simulink model "ESM_TeslaModelS_statKreisfahrt"  (R2020b)
settings: Solver=FixedStepAuto  StartTime=0.0  StopTime=StopTime  FixedStep=SampleTime  RelTol=1e-3
undefined symbols (not defined in the file): ayObs, c_alpha_F, c_alpha_R, c_alpha_rear_mean, DiscIntNeverNeededParam, I_S, init, input_r, m_vehicle, par_TIR, par_VEH, parameter, SelectManeuver, simtime, Single_Track_Model_linear, SingleTrackModel_linear
libraries: pid_lib x5, simulink x3, dspsigops x2, vehicle_model x1
(part 3 of 4)

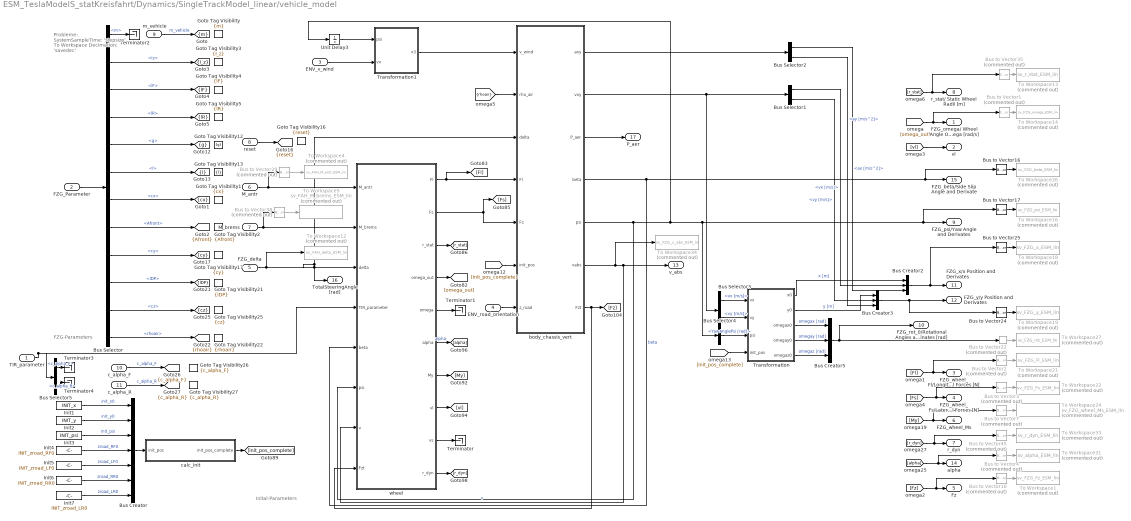
== system ESM_TeslaModelS_statKreisfahrt/Dynamics/SingleTrackModel_linear/vehicle_model ==
  note: Probleme:
      | SystemSampleTime: 'stepsize'
      |
      |
      | To Workspace
      | Decimation: 'savedec'
  note: FZG-Parameters
  note: Inital-Parameters
  TIR_parameter : Inport
  FZG_Parameter : Inport  Port=2
  ENV_v_wind : Inport  Port=3
  ENV_road_orientation : Inport  Port=4
  FZG_delta : Inport  Port=5
  M_antr : Inport  Port=6  PortDimensions=2
  M_brems : Inport  Port=7  PortDimensions=2
  reset : Inport  Port=8
  m_vehicle : Inport  Port=9
  c_alpha_F : Inport  Port=10
  c_alpha_R : Inport  Port=11
  Bus Creator : BusCreator  Inputs=7
  Bus Creator2 : BusCreator  Inputs=3
  Bus Creator3 : BusCreator  Inputs=3
  Bus Creator5 : BusCreator  Inputs=3
  Bus Selector : BusSelector  OutputSignals=m,Iz,lF,lR,g,l,cx,Afront,cy,lDP,cz,rhoair
  Bus Selector1 : BusSelector  OutputSignals=vx [m/s],vy [m/s]
  Bus Selector2 : BusSelector  OutputSignals=ax [m/s^2],ay [m/s^2]
  Bus Selector3 : BusSelector  OutputSignals=vx [m/s],vy [m/s]
  Bus Selector4 : BusSelector  OutputSignals=YawAnglePsi [rad]
  Bus Selector5 : BusSelector  OutputSignals=front.c_alpha_F,rear.c_alpha_R
  Bus to Vector{1..4,7,10,22,29,35,38,45} (11 alike) : BusToVector  Commented=on
  Bus to Vector{16..17,24..25} (4 alike) : BusToVector
  Goto Tag Visibility : GotoTagVisibility  GotoTag=m
  Goto Tag Visibility1 : GotoTagVisibility  GotoTag=cx
  Goto Tag Visibility12 : GotoTagVisibility  GotoTag=g
  Goto Tag Visibility13 : GotoTagVisibility  GotoTag=l
  Goto Tag Visibility16 : GotoTagVisibility  GotoTag=reset
  Goto Tag Visibility17 : GotoTagVisibility  GotoTag=cy
  Goto Tag Visibility2 : GotoTagVisibility  GotoTag=Afront
  Goto Tag Visibility21 : GotoTagVisibility  GotoTag=lDP
  Goto Tag Visibility22 : GotoTagVisibility  GotoTag=rhoair
  Goto Tag Visibility25 : GotoTagVisibility  GotoTag=cz
  Goto Tag Visibility26 : GotoTagVisibility  GotoTag=c_alpha_F
  Goto Tag Visibility27 : GotoTagVisibility  GotoTag=c_alpha_R
  Goto Tag Visibility3 : GotoTagVisibility  GotoTag=I_z
  Goto Tag Visibility4 : GotoTagVisibility  GotoTag=lF
  Goto Tag Visibility5 : GotoTagVisibility  GotoTag=lR
  Init1 : Constant  Value=INIT_x
  Init2 : Constant  Value=INIT_y
  Init3 : Constant  Value=INIT_psi
  Init4 : Constant  Value=INIT_zroad_RF0
  Init5 : Constant  Value=INIT_zroad_LF0
  Init6 : Constant  Value=INIT_zroad_RR0
  Init7 : Constant  Value=INIT_zroad_LR0
  Terminator{,1..4} (5 alike) : Terminator
  To Workspace1 : ToWorkspace  Commented=on  VariableName=sv_FZG_Fz_ESM_lin  SampleTime=-1
      settings: Decimation=savedec  Save2DSignal=2-D array (concatenate along first dimension)
  To Workspace12 : ToWorkspace  Commented=on  VariableName=sv_FAH_delta_ESM_lin  SampleTime=-1
      settings: Decimation=savedec  Save2DSignal=2-D array (concatenate along first dimension)
  To Workspace13 : ToWorkspace  Commented=on  VariableName=sv_r_stat_ESM_lin  SampleTime=-1
      settings: Decimation=savedec  Save2DSignal=2-D array (concatenate along first dimension)
  To Workspace14 : ToWorkspace  Commented=on  VariableName=sv_FZG_omega_ESM_lin  SampleTime=-1
      settings: Decimation=savedec  Save2DSignal=2-D array (concatenate along first dimension)
  To Workspace16 : ToWorkspace  Commented=on  VariableName=sv_FZG_psi_ESM_lin  SampleTime=-1
      settings: Decimation=savedec  Save2DSignal=2-D array (concatenate along first dimension)
  To Workspace18 : ToWorkspace  Commented=on  VariableName=sv_FZG_x_ESM_lin  SampleTime=-1
      settings: Decimation=savedec  Save2DSignal=2-D array (concatenate along first dimension)
  To Workspace19 : ToWorkspace  Commented=on  VariableName=sv_FZG_y_ESM_lin  SampleTime=-1
      settings: Decimation=savedec  Save2DSignal=2-D array (concatenate along first dimension)
  To Workspace21 : ToWorkspace  Commented=on  VariableName=sv_FZG_Fl_ESM_lin  SampleTime=-1
      settings: Decimation=savedec  Save2DSignal=2-D array (concatenate along first dimension)
  To Workspace22 : ToWorkspace  Commented=on  VariableName=sv_FZG_Fs_ESM_lin  SampleTime=-1
      settings: Decimation=savedec  Save2DSignal=2-D array (concatenate along first dimension)
  To Workspace24 : ToWorkspace  Commented=on  VariableName=sv_FZG_wheel_Ms_ESM_lin  SampleTime=-1
      settings: Decimation=savedec  Save2DSignal=2-D array (concatenate along first dimension)
  To Workspace26 : ToWorkspace  Commented=on  VariableName=sv_FZG_beta_ESM_lin  SampleTime=-1
      settings: Decimation=savedec  Save2DSignal=2-D array (concatenate along first dimension)
  To Workspace27 : ToWorkspace  Commented=on  VariableName=sv_FZG_rot_ESM_lin  SampleTime=-1
      settings: Decimation=savedec  Save2DSignal=2-D array (concatenate along first dimension)
  To Workspace31 : ToWorkspace  Commented=on  VariableName=sv_alpha_ESM_lin  SampleTime=-1
      settings: Decimation=savedec  Save2DSignal=2-D array (concatenate along first dimension)
  To Workspace33 : ToWorkspace  Commented=on  VariableName=sv_r_dyn_ESM_lin  SampleTime=-1
      settings: Decimation=savedec  Save2DSignal=2-D array (concatenate along first dimension)
  To Workspace34 : ToWorkspace  Commented=on  VariableName=sv_FZG_v_abs_ESM_lin  SampleTime=-1
      settings: Decimation=savedec  Save2DSignal=2-D array (concatenate along first dimension)
  To Workspace4 : ToWorkspace  Commented=on  VariableName=sv_FAH_M_antr_ESM_lin  SampleTime=-1
      settings: Decimation=savedec  Save2DSignal=2-D array (concatenate along first dimension)
  To Workspace5 : ToWorkspace  Commented=on  VariableName=sv_FAH_M_brems_ESM_lin  SampleTime=-1
      settings: Decimation=savedec  Save2DSignal=2-D array (concatenate along first dimension)
  Transformation : Subsystem
  Transformation1 : Subsystem
  Unit Delay3 : UnitDelay  SampleTime=-1  HasFrameUpgradeWarning=on
  body_chassis_vert : Subsystem
  calc_init : Subsystem
  wheel : Subsystem
  FZG_omega/ Wheel Angle Omega [rad/s] : Outport  VectorParamsAs1DForOutWhenUnconnected=off
  vl : Outport  Port=2  VectorParamsAs1DForOutWhenUnconnected=off
  FZG_wheel_Fl/Longitudinal Wheel Forces [N] : Outport  Port=3  VectorParamsAs1DForOutWhenUnconnected=off
  FZG_wheel_Fs/Lateral Wheel Forces [N] : Outport  Port=4  VectorParamsAs1DForOutWhenUnconnected=off
  Fz : Outport  Port=5  VectorParamsAs1DForOutWhenUnconnected=off
  FZG_wheel_Ms : Outport  Port=6  VectorParamsAs1DForOutWhenUnconnected=off
  r_dyn : Outport  Port=7  VectorParamsAs1DForOutWhenUnconnected=off
  r_stat/ Static Wheel Radii [m] : Outport  Port=8  VectorParamsAs1DForOutWhenUnconnected=off
  FZG_psi/Yaw Angle and Derivates : Outport  Port=9  VectorParamsAs1DForOutWhenUnconnected=off
  FZG_rot_0/Rotational Angles around Initial Coordinates [rad] : Outport  Port=10  VectorParamsAs1DForOutWhenUnconnected=off
  FZG_x/x Position and Derivates : Outport  Port=11  PortDimensions=3  VectorParamsAs1DForOutWhenUnconnected=off
  FZG_y/y Position and Derivates : Outport  Port=12  VectorParamsAs1DForOutWhenUnconnected=off
  v_abs : Outport  Port=13  VectorParamsAs1DForOutWhenUnconnected=off
  alpha : Outport  Port=14  VectorParamsAs1DForOutWhenUnconnected=off
  FZG_beta/Side Slip Angle and Derivate : Outport  Port=15  VectorParamsAs1DForOutWhenUnconnected=off
  TotalSteeringAngle [rad] : Outport  Port=16  VectorParamsAs1DForOutWhenUnconnected=off
  P_aer : Outport  Port=17  VectorParamsAs1DForOutWhenUnconnected=off
  tag scope: Afront=scoped, I_z=scoped, c_alpha_F=scoped, c_alpha_R=scoped, cx=scoped, cy=scoped, cz=scoped, g=scoped, l=scoped, lDP=scoped, lF=scoped, lR=scoped, m=scoped, reset=scoped, rhoair=scoped
  wires:
  M_antr/1 -> wheel/1(M_antr), Bus to Vector29/1
  Bus to Vector29/1 -> To Workspace4/1
  M_brems/1 -> Bus to Vector38/1, wheel/2(M_brems)
  Bus to Vector38/1 -> To Workspace5/1
  FZG_delta/1 -> wheel/3(delta), body_chassis_vert/3(delta), TotalSteeringAngle [rad]/1, To Workspace12/1
  Bus to Vector2/1 -> To Workspace21/1
  Bus to Vector25/1 -> To Workspace18/1
  Bus Creator5/1 -> Bus to Vector22/1, FZG_rot_0/Rotational Angles around Initial Coordinates [rad]/1
  Bus to Vector4/1 -> To Workspace31/1
  Bus to Vector1/1 -> To Workspace14/1
  Bus to Vector16/1 -> To Workspace26/1
  Bus to Vector24/1 -> To Workspace19/1
  [omega_out] -> FZG_omega/ Wheel Angle Omega [rad/s]/1, Bus to Vector1/1
  Bus to Vector17/1 -> To Workspace16/1
  Bus Creator3/1 -> Bus to Vector24/1, FZG_y/y Position and Derivates/1
  Bus to Vector3/1 -> To Workspace22/1
  Bus to Vector7/1 -> To Workspace24/1
  Bus to Vector35/1 -> To Workspace13/1
  Bus to Vector45/1 -> To Workspace33/1
  [Fl] -> FZG_wheel_Fl/Longitudinal Wheel Forces [N]/1, Bus to Vector2/1
  body_chassis_vert/5(psi) -> wheel/6(psi), Unit Delay3/1, Bus Selector4/1, FZG_psi/Yaw Angle and Derivates/1, Bus to Vector17/1
  [Fs] -> FZG_wheel_Fs/Lateral Wheel Forces [N]/1, Bus to Vector3/1
  [r_dyn] -> r_dyn/1, Bus to Vector45/1
  [My] -> FZG_wheel_Ms/1, Bus to Vector7/1
  Bus to Vector10/1 -> To Workspace1/1
  body_chassis_vert/4(beta) -> wheel/5(beta), FZG_beta/Side Slip Angle and Derivate/1, Bus to Vector16/1  "beta"
  [Fz] -> Fz/1, Bus to Vector10/1
  Bus Creator2/1 -> FZG_x/x Position and Derivates/1, Bus to Vector25/1
  [r_stat] -> r_stat/ Static Wheel Radii [m]/1, Bus to Vector35/1
  [alpha] -> alpha/1, Bus to Vector4/1
  Bus to Vector22/1 -> To Workspace27/1
  c_alpha_R/1 -> [c_alpha_R]  "c_alpha_R"
  c_alpha_F/1 -> [c_alpha_F]  "c_alpha_F"
  Init7/1 -> Bus Creator/7  "zroad_LR0"
  Init6/1 -> Bus Creator/6  "zroad_RR0"
  Init5/1 -> Bus Creator/5  "zroad_LF0"
  Init4/1 -> Bus Creator/4  "zroad_RF0"
  Init3/1 -> Bus Creator/3  "init_psi"
  Init2/1 -> Bus Creator/2  "init_y0"
  Init1/1 -> Bus Creator/1  "init_x0"
  [vl] -> vl/1
  wheel/10(r_dyn) -> [r_dyn]
  wheel/6(alpha) -> [alpha]  "alpha"
  wheel/9(vs) -> Terminator/1
  wheel/8(vl) -> [vl]
  wheel/7(My) -> [My]
  wheel/3(r_stat) -> [r_stat]
  [init_pos_complete] -> Transformation/4(init_pos)
  [init_pos_complete] -> body_chassis_vert/6(init_pos)
  calc_init/1(init_pos_complete) -> [init_pos_complete]
  TIR_parameter/1 -> wheel/4(TIR_parameter), Bus Selector5/1
  wheel/5(omega) -> Terminator1/1
  wheel/4(omega_out) -> [omega_out]
  body_chassis_vert/3(P_aer) -> P_aer/1
  Bus Selector/7 -> [cx]  "<cx>"
  Bus Selector/8 -> [Afront]  "<Afront>"
  Bus Selector/10 -> [lDP]  "<lDP>"
  Bus Selector/11 -> [cz]  "<cz>"
  body_chassis_vert/1(axy) -> Bus Selector2/1
  body_chassis_vert/2(vxy) -> Bus Selector1/1, Bus Selector3/1
  Bus Selector/9 -> [cy]  "<cy>"
  Unit Delay3/1 -> Transformation1/1(psi)
  Transformation1/1(x3) -> body_chassis_vert/1(v_wind)
  Bus Creator/1 -> calc_init/1(init_pos)
  Transformation/5(omegaz0) -> Bus Creator5/3  "omegaz [rad]"
  Transformation/4(omegay0) -> Bus Creator5/2  "omegay [rad]"
  Transformation/3(omegax0) -> Bus Creator5/1  "omegax [rad]"
  Bus Selector4/1 -> Transformation/3(psi)  "<YawAnglePsi [rad]>"
  Bus Selector3/2 -> Transformation/2(vy)  "<vy [m/s]>"
  Bus Selector3/1 -> Transformation/1(vx)  "<vx [m/s]>"
  Transformation/2(y0) -> Bus Creator3/1  "y [m]"
  Transformation/1(x0) -> Bus Creator2/1  "x [m]"
  ENV_road_orientation/1 -> body_chassis_vert/7(z_road)
  [rhoair] -> body_chassis_vert/2(rho_air)
  ENV_v_wind/1 -> Transformation1/2(vx)
  FZG_Parameter/1 -> Bus Selector/1
  wheel/2(Fs) -> body_chassis_vert/5(Fs), [Fs]
  body_chassis_vert/6(vabs) -> wheel/7(v), v_abs/1, To Workspace34/1  "v"
  Bus Selector/1 -> Terminator2/1  "<m>"
  Bus Selector/2 -> [I_z]  "<Iz>"
  Bus Selector/3 -> [lF]  "<lF>"
  Bus Selector/4 -> [lR]  "<lR>"
  Bus Selector/5 -> [g]  "<g>"
  Bus Selector/6 -> [l]  "<l>"
  wheel/1(Fl) -> body_chassis_vert/4(Fl), [Fl]
  Bus Selector1/1 -> Bus Creator2/2  "<vx [m/s]>"
  Bus Selector1/2 -> Bus Creator3/2  "<vy [m/s]>"
  Bus Selector2/1 -> Bus Creator2/3  "<ax [m/s^2]>"
  Bus Selector2/2 -> Bus Creator3/3  "<ay [m/s^2]>"
  reset/1 -> [reset]
  body_chassis_vert/7(Fzt) -> [Fz], wheel/8(Fzt)
  Bus Selector/12 -> [rhoair]  "<rhoair>"
  m_vehicle/1 -> [m]  "m_vehicle"
  Bus Selector5/2 -> Terminator4/1  "<c_alpha_R>"
  Bus Selector5/1 -> Terminator3/1  "<c_alpha_F>"

== system ESM_TeslaModelS_statKreisfahrt/Driver and Environment/quasistationare Kreisfahrt/PID Driver Steering r/driver ==
  note: I-Glied muss proportional an stepsize angepasst werden.
      | Gute Einstellung: Stepsize 0.0005 , I-Glied: 100 , P-Glied: 0
  r ist : Inport
  r soll : Inport  Port=2
  Math Function : Math  Operator=reciprocal  SignedPower=on  SaturateOnIntegerOverflow=on
  Math Function1 : Math  Operator=reciprocal  SignedPower=on  SaturateOnIntegerOverflow=on
  PI-Controller : Subsystem
  Sum1 : Sum  Inputs=|-+
  not_zero : Subsystem
  not_zero1 : Subsystem
  delta_h : Outport  VectorParamsAs1DForOutWhenUnconnected=off
  wires:
  r soll/1 -> not_zero1/1(In1)
  r ist/1 -> not_zero/1(In1)
  not_zero1/1(Out1) -> Math Function1/1
  not_zero/1(Out1) -> Math Function/1
  Sum1/1 -> PI-Controller/1(" Regelabweichung")
  Math Function1/1 -> Sum1/2
  Math Function/1 -> Sum1/1
  PI-Controller/1(Stellgröße) -> delta_h/1

== system ESM_TeslaModelS_statKreisfahrt/Driver and Environment/quasistationare Kreisfahrt/PID Driver Steering r/not_zero ==
  In1 : Inport
  Constant : Constant  Value=0.0000000000001
  Switch : Switch  Criteria=u2 ~= 0  Threshold=0.1
  Out1 : Outport  VectorParamsAs1DForOutWhenUnconnected=off
  wires:
  In1/1 -> Switch/1, Switch/2
  Constant/1 -> Switch/3
  Switch/1 -> Out1/1

== system ESM_TeslaModelS_statKreisfahrt/Driver and Environment/quasistationare Kreisfahrt mit Lastwechsel Beschleunigung/PID Driver Steering r_mit Lastwechsel Beschleunigung/driver ==
  note: I-Glied muss proportional an stepsize angepasst werden.
      | Gute Einstellung: Stepsize 0.0005 , I-Glied: 100 , P-Glied: 0
  r ist : Inport
  r soll : Inport  Port=2
  Math Function2 : Math  Operator=reciprocal  SignedPower=on  SaturateOnIntegerOverflow=on
  Math Function3 : Math  Operator=reciprocal  SignedPower=on  SaturateOnIntegerOverflow=on
  PI-Controller : Subsystem
  Sample and Hold : dspsigops/Sample and Hold  trig=Falling edge  initCond=0  latchinput=off
  Step1 : Step  Time=153  Before=1  After=0  SampleTime=0
  Sum2 : Sum  Inputs=|-+
  Switch1 : Switch  Criteria=u2 > Threshold
  not_zero2 : Subsystem
  not_zero3 : Subsystem
  delta_h : Outport  VectorParamsAs1DForOutWhenUnconnected=off
  wires:
  Math Function2/1 -> Sum2/1
  Sum2/1 -> PI-Controller/1(" Regelabweichung")
  Math Function3/1 -> Sum2/2
  not_zero3/1(Out1) -> Math Function3/1
  r ist/1 -> not_zero2/1(In1)
  not_zero2/1(Out1) -> Math Function2/1
  r soll/1 -> not_zero3/1(In1)
  Switch1/1 -> delta_h/1
  Step1/1 -> Sample and Hold/Trigger, Switch1/2
  PI-Controller/1(Stellgröße) -> Sample and Hold/1, Switch1/1
  Sample and Hold/1 -> Switch1/3

== system ESM_TeslaModelS_statKreisfahrt/Driver and Environment/quasistationare Kreisfahrt mit Lastwechsel Beschleunigung/PID Driver Steering r_mit Lastwechsel Beschleunigung/not_zero ==
  In1 : Inport
  Constant : Constant  Value=0.0000000000001
  Switch : Switch  Criteria=u2 ~= 0
  Out1 : Outport  VectorParamsAs1DForOutWhenUnconnected=off
  wires:
  In1/1 -> Switch/1, Switch/2
  Constant/1 -> Switch/3
  Switch/1 -> Out1/1

== system ESM_TeslaModelS_statKreisfahrt/Driver and Environment/quasistationare Kreisfahrt mit Lastwechsel Verzogerung/PID Driver Steering r_mit Lastwechsel Verzogerung/driver ==
  note: I-Glied muss proportional an stepsize angepasst werden.
      | Gute Einstellung: Stepsize 0.0005 , I-Glied: 100 , P-Glied: 0
  r ist : Inport
  r soll : Inport  Port=2
  Math Function2 : Math  Operator=reciprocal  SignedPower=on  SaturateOnIntegerOverflow=on
  Math Function3 : Math  Operator=reciprocal  SignedPower=on  SaturateOnIntegerOverflow=on
  PI-Controller : Subsystem
  Sample and Hold : dspsigops/Sample and Hold  trig=Falling edge  initCond=0  latchinput=off
  Step1 : Step  Time=0.9799  Before=1  After=0  SampleTime=0
  Sum2 : Sum  Inputs=|-+
  Switch1 : Switch  Criteria=u2 > Threshold
  not_zero2 : Subsystem
  not_zero3 : Subsystem
  delta_h : Outport  VectorParamsAs1DForOutWhenUnconnected=off
  wires:
  Sample and Hold/1 -> Switch1/3
  PI-Controller/1(Stellgröße) -> Switch1/1, Sample and Hold/1
  Step1/1 -> Switch1/2, Sample and Hold/Trigger
  Switch1/1 -> delta_h/1
  r soll/1 -> not_zero3/1(In1)
  not_zero2/1(Out1) -> Math Function2/1
  r ist/1 -> not_zero2/1(In1)
  not_zero3/1(Out1) -> Math Function3/1
  Math Function3/1 -> Sum2/2
  Sum2/1 -> PI-Controller/1(" Regelabweichung")
  Math Function2/1 -> Sum2/1

== system ESM_TeslaModelS_statKreisfahrt/Driver and Environment/quasistationare Kreisfahrt mit Lastwechsel Verzogerung/PID Driver Steering r_mit Lastwechsel Verzogerung/not_zero ==
  In1 : Inport
  Constant : Constant  Value=0.0000000000001
  Switch : Switch  Criteria=u2 ~= 0
  Out1 : Outport  VectorParamsAs1DForOutWhenUnconnected=off
  wires:
  Switch/1 -> Out1/1
  Constant/1 -> Switch/3
  In1/1 -> Switch/2, Switch/1

== system ESM_TeslaModelS_statKreisfahrt/Dynamics/SingleTrackModel_linear/Tire_Parameters/param_tire_model ==
  note: TIRE DATA
  note: TIRE DATA
  Bus Creator : BusCreator  Inputs=2
  Bus Creator2 : BusCreator  Inputs=2
  Bus Creator4 : BusCreator  Inputs=2
  Constant : Constant  Value=par_TIR(2).unloadedRadius
  Constant1 : Constant  Value=par_TIR(1).c_alpha_F
  Constant137 : Constant  Value=par_TIR(1).unloadedRadius
  Constant2 : Constant  Value=par_TIR(2).c_alpha_R
  TIR_parameter : Outport  VectorParamsAs1DForOutWhenUnconnected=off
  wires:
  Constant2/1 -> Bus Creator/2  "c_alpha_R"
  Constant1/1 -> Bus Creator2/2  "c_alpha_F"
  Constant137/1 -> Bus Creator2/1  "UNLOADED_RADIUS"
  Constant/1 -> Bus Creator/1  "UNLOADED_RADIUS"
  Bus Creator/1 -> Bus Creator4/2  "rear"
  Bus Creator2/1 -> Bus Creator4/1  "front"
  Bus Creator4/1 -> TIR_parameter/1

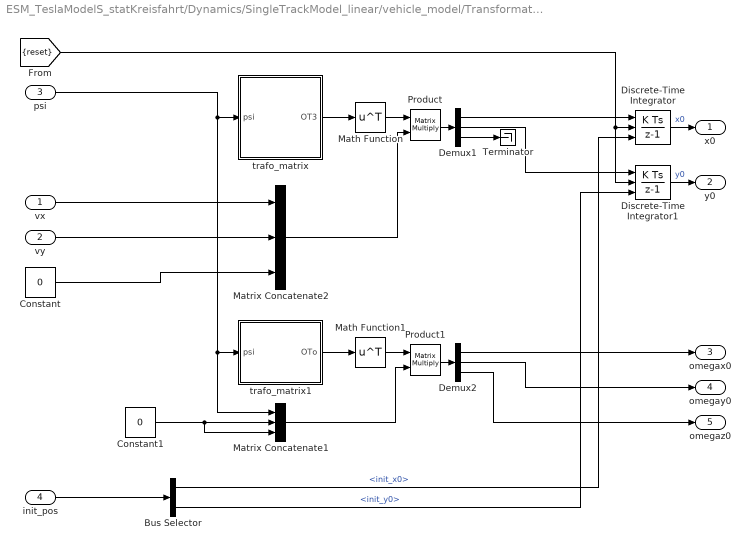
== system ESM_TeslaModelS_statKreisfahrt/Dynamics/SingleTrackModel_linear/vehicle_model/Transformation ==
  vx : Inport
  vy : Inport  Port=2
  psi : Inport  Port=3
  init_pos : Inport  Port=4
  Bus Selector : BusSelector  OutputSignals=init_x0,init_y0
  Constant : Constant  Value=0
  Constant1 : Constant  Value=0
  Demux1 : Demux  Outputs=3
  Demux2 : Demux  Outputs=3
  Discrete-Time Integrator : DiscreteIntegrator  ExternalReset=sampled level  InitialConditionSource=external  SampleTime=-1  ICPrevOutput=DiscIntNeverNeededParam  ICPrevScaledInput=DiscIntNeverNeededParam
  Discrete-Time Integrator1 : DiscreteIntegrator  ExternalReset=sampled level  InitialConditionSource=external  SampleTime=-1  ICPrevOutput=DiscIntNeverNeededParam  ICPrevScaledInput=DiscIntNeverNeededParam
  Math Function : Math  Operator=transpose  SignedPower=on  SaturateOnIntegerOverflow=on
  Math Function1 : Math  Operator=transpose  SignedPower=on  SaturateOnIntegerOverflow=on
  Matrix Concatenate1 : Concatenate  NumInputs=3
  Matrix Concatenate2 : Concatenate  NumInputs=3
  Product : Product  Multiplication=Matrix(*)
  Product1 : Product  Multiplication=Matrix(*)
  Terminator : Terminator
  trafo_matrix : Subsystem
  trafo_matrix1 : Subsystem
  x0 : Outport  VectorParamsAs1DForOutWhenUnconnected=off
  y0 : Outport  Port=2  VectorParamsAs1DForOutWhenUnconnected=off
  omegax0 : Outport  Port=3  VectorParamsAs1DForOutWhenUnconnected=off
  omegay0 : Outport  Port=4  VectorParamsAs1DForOutWhenUnconnected=off
  omegaz0 : Outport  Port=5  VectorParamsAs1DForOutWhenUnconnected=off
  wires:
  Product1/1 -> Demux2/1
  trafo_matrix1/1(OTo) -> Math Function1/1
  Math Function1/1 -> Product1/1
  Matrix Concatenate1/1 -> Product1/2
  Product/1 -> Demux1/1
  Demux1/3 -> Terminator/1
  Math Function/1 -> Product/1
  Constant/1 -> Matrix Concatenate2/3
  Matrix Concatenate2/1 -> Product/2
  trafo_matrix/1(OT3) -> Math Function/1
  Bus Selector/2 -> Discrete-Time Integrator1/3  "<init_y0>"
  Bus Selector/1 -> Discrete-Time Integrator/3  "<init_x0>"
  init_pos/1 -> Bus Selector/1
  Demux2/3 -> omegaz0/1
  Demux2/2 -> omegay0/1
  Demux2/1 -> omegax0/1
  Discrete-Time Integrator1/1 -> y0/1  "y0"
  Discrete-Time Integrator/1 -> x0/1  "x0"
  vy/1 -> Matrix Concatenate2/2
  vx/1 -> Matrix Concatenate2/1
  psi/1 -> trafo_matrix1/1(psi), Matrix Concatenate1/1, trafo_matrix/1(psi)
  Demux1/2 -> Discrete-Time Integrator1/1
  Demux1/1 -> Discrete-Time Integrator/1
  [reset] -> Discrete-Time Integrator/2, Discrete-Time Integrator1/2
  Constant1/1 -> Matrix Concatenate1/3, Matrix Concatenate1/2

== system ESM_TeslaModelS_statKreisfahrt/Dynamics/SingleTrackModel_linear/vehicle_model/Transformation1 ==
  psi : Inport
  vx : Inport  Port=2
  Bus Creator : BusCreator  Inputs=3
  Bus Selector : BusSelector  OutputSignals=vx,vy,vz
  Bus Selector1 : BusSelector  OutputSignals=YawAnglePsi [rad]
  Demux1 : Demux  Outputs=3
  Math Function : Math  Operator=transpose  SignedPower=on  SaturateOnIntegerOverflow=on
  Matrix Concatenate2 : Concatenate  NumInputs=3
  Product : Product  Multiplication=Matrix(*)
  trafo_matrix : Subsystem
  x3 : Outport  VectorParamsAs1DForOutWhenUnconnected=off
  wires:
  Product/1 -> Demux1/1
  Math Function/1 -> Product/1
  Matrix Concatenate2/1 -> Product/2
  trafo_matrix/1(OT3) -> Math Function/1
  psi/1 -> Bus Selector1/1
  Demux1/3 -> Bus Creator/3  "vwindz"
  Demux1/2 -> Bus Creator/2  "vwindy"
  Demux1/1 -> Bus Creator/1  "vwindx"
  Bus Selector/3 -> Matrix Concatenate2/3  "<vz>"
  Bus Selector/2 -> Matrix Concatenate2/2  "<vy>"
  Bus Selector/1 -> Matrix Concatenate2/1  "<vx>"
  vx/1 -> Bus Selector/1
  Bus Creator/1 -> x3/1
  Bus Selector1/1 -> trafo_matrix/1(psi)  "<YawAnglePsi [rad]>"

== system ESM_TeslaModelS_statKreisfahrt/Dynamics/SingleTrackModel_linear/vehicle_model/body_chassis_vert ==
  v_wind : Inport
  rho_air : Inport  Port=2
  delta : Inport  Port=3
  Fl : Inport  Port=4
  Fs : Inport  Port=5
  init_pos : Inport  Port=6
  z_road : Inport  Port=7
  horizontal : Subsystem
  road_orientation : Subsystem
  transformation : Subsystem
  vertical : Subsystem
  axy : Outport  VectorParamsAs1DForOutWhenUnconnected=off
  vxy : Outport  Port=2  VectorParamsAs1DForOutWhenUnconnected=off
  P_aer : Outport  Port=3  VectorParamsAs1DForOutWhenUnconnected=off
  beta : Outport  Port=4  VectorParamsAs1DForOutWhenUnconnected=off
  psi : Outport  Port=5  VectorParamsAs1DForOutWhenUnconnected=off
  vabs : Outport  Port=6  VectorParamsAs1DForOutWhenUnconnected=off
  Fzt : Outport  Port=7  VectorParamsAs1DForOutWhenUnconnected=off
  wires:
  road_orientation/1(theta_road) -> horizontal/7(pitch_road)
  z_road/1 -> road_orientation/1(zroad)
  horizontal/6(vx) -> transformation/3(vx)  "vx"
  horizontal/7(vy) -> transformation/4(vy)  "vy"
  horizontal/5(ay) -> transformation/2(ay)  "ay"
  horizontal/4(ax) -> transformation/1(ax)  "ax"
  transformation/1(axy) -> axy/1
  transformation/2(vxy) -> vxy/1
  v_wind/1 -> horizontal/6(v_wind)
  init_pos/1 -> horizontal/5(init_pos)
  rho_air/1 -> horizontal/4(rho_air)
  delta/1 -> horizontal/1(delta)
  horizontal/1(beta) -> beta/1
  horizontal/2(psi) -> psi/1
  Fl/1 -> horizontal/2(Fl)
  horizontal/3(v_abs) -> vabs/1
  Fs/1 -> horizontal/3(Fs)
  horizontal/8(P_aer) -> P_aer/1
  vertical/1(F_vert) -> Fzt/1

== system ESM_TeslaModelS_statKreisfahrt/Dynamics/SingleTrackModel_linear/vehicle_model/calc_init ==
  init_pos : Inport
  Bus Creator : BusCreator  Inputs=9
  Bus Selector : BusSelector  OutputSignals=init_x0,init_y0,init_psi,zroad_RF0,zroad_LF0,zroad_RR0,zroad_LR0
  pitch : Subsystem
  vertical : Subsystem
  init_pos_complete : Outport  VectorParamsAs1DForOutWhenUnconnected=off
  wires:
  Bus Creator/1 -> init_pos_complete/1
  vertical/1(init_z0) -> Bus Creator/9  "init_z0"
  Bus Selector/7 -> Bus Creator/7  "<zroad_LR0>"
  Bus Selector/6 -> Bus Creator/6  "<zroad_RR0>"
  Bus Selector/5 -> Bus Creator/5  "<zroad_LF0>"
  Bus Selector/4 -> Bus Creator/4  "<zroad_RF0>"
  Bus Selector/3 -> Bus Creator/3  "<init_psi>"
  Bus Selector/2 -> Bus Creator/2  "<init_y0>"
  Bus Selector/1 -> Bus Creator/1  "<init_x0>"
  pitch/1(init_theta) -> vertical/2(theta), Bus Creator/8  "init_theta"
  init_pos/1 -> Bus Selector/1, vertical/1(init_pos), pitch/1(init_pos)

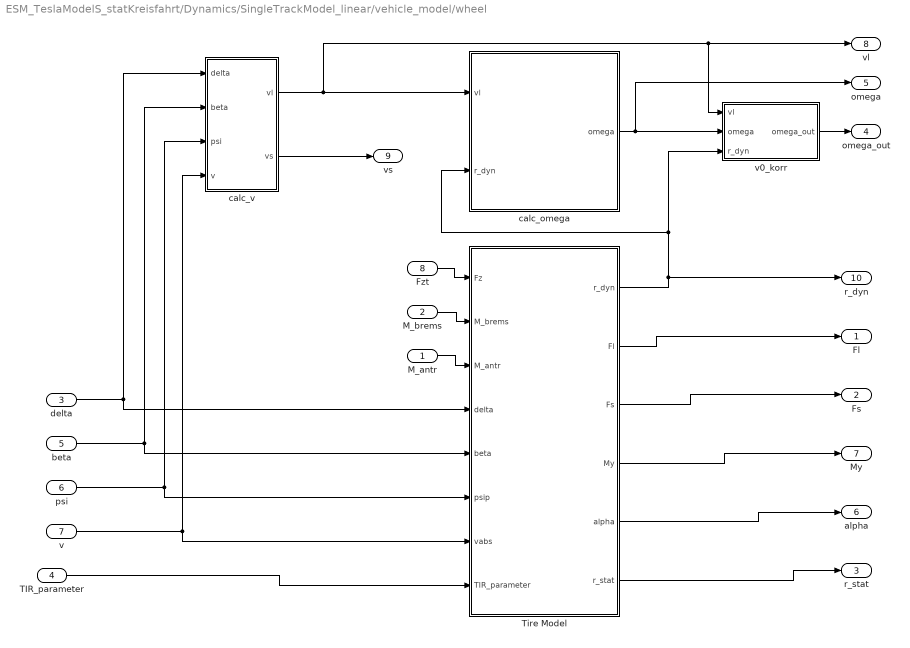
== system ESM_TeslaModelS_statKreisfahrt/Dynamics/SingleTrackModel_linear/vehicle_model/wheel ==
  M_antr : Inport
  M_brems : Inport  Port=2
  delta : Inport  Port=3
  TIR_parameter : Inport  Port=4
  beta : Inport  Port=5
  psi : Inport  Port=6
  v : Inport  Port=7
  Fzt : Inport  Port=8
  Tire Model : Subsystem
  calc_omega : Subsystem
  calc_v : Subsystem
  v0_korr : Subsystem
  Fl : Outport  VectorParamsAs1DForOutWhenUnconnected=off
  Fs : Outport  Port=2  VectorParamsAs1DForOutWhenUnconnected=off
  r_stat : Outport  Port=3  VectorParamsAs1DForOutWhenUnconnected=off
  omega_out : Outport  Port=4  VectorParamsAs1DForOutWhenUnconnected=off
  omega : Outport  Port=5  VectorParamsAs1DForOutWhenUnconnected=off
  alpha : Outport  Port=6  VectorParamsAs1DForOutWhenUnconnected=off
  My : Outport  Port=7  VectorParamsAs1DForOutWhenUnconnected=off
  vl : Outport  Port=8  VectorParamsAs1DForOutWhenUnconnected=off
  vs : Outport  Port=9  VectorParamsAs1DForOutWhenUnconnected=off
  r_dyn : Outport  Port=10  VectorParamsAs1DForOutWhenUnconnected=off
  wires:
  M_brems/1 -> Tire Model/2(M_brems)
  Tire Model/1(r_dyn) -> v0_korr/3(r_dyn), calc_omega/2(r_dyn), r_dyn/1
  Tire Model/6(r_stat) -> r_stat/1
  v0_korr/1(omega_out) -> omega_out/1
  Tire Model/2(Fl) -> Fl/1
  Tire Model/4(My) -> My/1
  calc_omega/1(omega) -> omega/1, v0_korr/2(omega)
  calc_v/1(vl) -> calc_omega/1(vl), vl/1, v0_korr/1(vl)
  calc_v/2(vs) -> vs/1
  delta/1 -> calc_v/1(delta), Tire Model/4(delta)
  psi/1 -> calc_v/3(psi), Tire Model/6(psip)
  beta/1 -> calc_v/2(beta), Tire Model/5(beta)
  M_antr/1 -> Tire Model/3(M_antr)
  Tire Model/3(Fs) -> Fs/1
  TIR_parameter/1 -> Tire Model/8(TIR_parameter)
  Tire Model/5(alpha) -> alpha/1
  v/1 -> calc_v/4(v), Tire Model/7(vabs)
  Fzt/1 -> Tire Model/1(Fz)

== system ESM_TeslaModelS_statKreisfahrt/Driver and Environment/quasistationare Kreisfahrt/PID Driver Steering r/driver/PI-Controller ==
  " Regelabweichung" : Inport
  Discrete-Time Integrator : DiscreteIntegrator  gainval=1  SampleTime=-1  LimitOutput=on  UpperSaturationLimit=1  LowerSaturationLimit=-1  ICPrevOutput=DiscIntNeverNeededParam  ICPrevScaledInput=DiscIntNeverNeededParam
  Gain : Gain  Gain=P_S  ParamDataTypeStr=double
  I-Glied : Gain  Gain=I_S  ParamDataTypeStr=double
  Saturation1 : Saturate  UpperLimit=0.6  LowerLimit=-0.6
  Signal Specification : SignalSpecification  OutDataTypeStr=double  Dimensions=1
  Sum2 : Sum  Inputs=|++
  Stellgröße : Outport  VectorParamsAs1DForOutWhenUnconnected=off
  wires:
  Discrete-Time Integrator/1 -> Sum2/2
  Saturation1/1 -> Stellgröße/1
  Gain/1 -> Signal Specification/1
  Signal Specification/1 -> Sum2/1
  Sum2/1 -> Saturation1/1
  " Regelabweichung"/1 -> I-Glied/1, Gain/1
  I-Glied/1 -> Discrete-Time Integrator/1

== system ESM_TeslaModelS_statKreisfahrt/Driver and Environment/quasistationare Kreisfahrt/PID Driver Steering r/driver/not_zero ==
  In1 : Inport
  Constant : Constant  Value=0.0000000000001
  Switch : Switch  Criteria=u2 ~= 0
  Out1 : Outport  VectorParamsAs1DForOutWhenUnconnected=off
  wires:
  In1/1 -> Switch/1, Switch/2
  Constant/1 -> Switch/3
  Switch/1 -> Out1/1

== system ESM_TeslaModelS_statKreisfahrt/Driver and Environment/quasistationare Kreisfahrt/PID Driver Steering r/driver/not_zero1 ==
  In1 : Inport
  Constant : Constant  Value=0.0000000000001
  Switch : Switch  Criteria=u2 ~= 0
  Out1 : Outport  VectorParamsAs1DForOutWhenUnconnected=off
  wires:
  Switch/1 -> Out1/1
  Constant/1 -> Switch/3
  In1/1 -> Switch/2, Switch/1

== system ESM_TeslaModelS_statKreisfahrt/Driver and Environment/quasistationare Kreisfahrt mit Lastwechsel Beschleunigung/PID Driver Steering r_mit Lastwechsel Beschleunigung/driver/PI-Controller ==
  " Regelabweichung" : Inport
  Discrete-Time Integrator : DiscreteIntegrator  gainval=1  SampleTime=-1  LimitOutput=on  UpperSaturationLimit=1  LowerSaturationLimit=-1  ICPrevOutput=DiscIntNeverNeededParam  ICPrevScaledInput=DiscIntNeverNeededParam
  Gain : Gain  Gain=P_S  ParamDataTypeStr=double
  I-Glied : Gain  Gain=I_S  ParamDataTypeStr=double
  Saturation1 : Saturate  UpperLimit=0.6  LowerLimit=-0.6
  Signal Specification : SignalSpecification  OutDataTypeStr=double  Dimensions=1
  Sum2 : Sum  Inputs=|++
  Stellgröße : Outport  VectorParamsAs1DForOutWhenUnconnected=off
  wires:
  I-Glied/1 -> Discrete-Time Integrator/1
  " Regelabweichung"/1 -> Gain/1, I-Glied/1
  Sum2/1 -> Saturation1/1
  Signal Specification/1 -> Sum2/1
  Gain/1 -> Signal Specification/1
  Saturation1/1 -> Stellgröße/1
  Discrete-Time Integrator/1 -> Sum2/2

== system ESM_TeslaModelS_statKreisfahrt/Driver and Environment/quasistationare Kreisfahrt mit Lastwechsel Beschleunigung/PID Driver Steering r_mit Lastwechsel Beschleunigung/driver/not_zero2 ==
  In1 : Inport
  Constant : Constant  Value=0.0000000000001
  Switch : Switch  Criteria=u2 ~= 0
  Out1 : Outport  VectorParamsAs1DForOutWhenUnconnected=off
  wires:
  Switch/1 -> Out1/1
  Constant/1 -> Switch/3
  In1/1 -> Switch/2, Switch/1

== system ESM_TeslaModelS_statKreisfahrt/Driver and Environment/quasistationare Kreisfahrt mit Lastwechsel Beschleunigung/PID Driver Steering r_mit Lastwechsel Beschleunigung/driver/not_zero3 ==
  In1 : Inport
  Constant : Constant  Value=0.0000000000001
  Switch : Switch  Criteria=u2 ~= 0
  Out1 : Outport  VectorParamsAs1DForOutWhenUnconnected=off
  wires:
  In1/1 -> Switch/1, Switch/2
  Constant/1 -> Switch/3
  Switch/1 -> Out1/1

== system ESM_TeslaModelS_statKreisfahrt/Driver and Environment/quasistationare Kreisfahrt mit Lastwechsel Verzogerung/PID Driver Steering r_mit Lastwechsel Verzogerung/driver/PI-Controller ==
  " Regelabweichung" : Inport
  Discrete-Time Integrator : DiscreteIntegrator  gainval=1  SampleTime=-1  LimitOutput=on  UpperSaturationLimit=1  LowerSaturationLimit=-1  ICPrevOutput=DiscIntNeverNeededParam  ICPrevScaledInput=DiscIntNeverNeededParam
  Gain : Gain  Gain=P_S  ParamDataTypeStr=double
  I-Glied : Gain  Gain=I_S  ParamDataTypeStr=double
  Saturation1 : Saturate  UpperLimit=0.6  LowerLimit=-0.6
  Signal Specification : SignalSpecification  OutDataTypeStr=double  Dimensions=1
  Sum2 : Sum  Inputs=|++
  Stellgröße : Outport  VectorParamsAs1DForOutWhenUnconnected=off
  wires:
  Discrete-Time Integrator/1 -> Sum2/2
  Saturation1/1 -> Stellgröße/1
  Gain/1 -> Signal Specification/1
  Signal Specification/1 -> Sum2/1
  Sum2/1 -> Saturation1/1
  " Regelabweichung"/1 -> I-Glied/1, Gain/1
  I-Glied/1 -> Discrete-Time Integrator/1

== system ESM_TeslaModelS_statKreisfahrt/Driver and Environment/quasistationare Kreisfahrt mit Lastwechsel Verzogerung/PID Driver Steering r_mit Lastwechsel Verzogerung/driver/not_zero2 ==
  In1 : Inport
  Constant : Constant  Value=0.0000000000001
  Switch : Switch  Criteria=u2 ~= 0
  Out1 : Outport  VectorParamsAs1DForOutWhenUnconnected=off
  wires:
  In1/1 -> Switch/1, Switch/2
  Constant/1 -> Switch/3
  Switch/1 -> Out1/1

== system ESM_TeslaModelS_statKreisfahrt/Driver and Environment/quasistationare Kreisfahrt mit Lastwechsel Verzogerung/PID Driver Steering r_mit Lastwechsel Verzogerung/driver/not_zero3 ==
  In1 : Inport
  Constant : Constant  Value=0.0000000000001
  Switch : Switch  Criteria=u2 ~= 0
  Out1 : Outport  VectorParamsAs1DForOutWhenUnconnected=off
  wires:
  Switch/1 -> Out1/1
  Constant/1 -> Switch/3
  In1/1 -> Switch/2, Switch/1

== system ESM_TeslaModelS_statKreisfahrt/Dynamics/SingleTrackModel_linear/vehicle_model/Transformation/trafo_matrix ==
  psi : Inport
  Constant{,2..4} (4 alike) : Constant  Value=0
  Constant1 : Constant
  Matrix Concatenate : Concatenate  NumInputs=3  Mode=Multidimensional array  ConcatenateDimension=2
  Matrix Concatenate1 : Concatenate  NumInputs=3
  Matrix Concatenate2 : Concatenate  NumInputs=3
  Matrix Concatenate3 : Concatenate  NumInputs=3
  Trigonometric Function : Trigonometry  Operator=cos
  Trigonometric Function7 : Trigonometry
  Unary Minus : UnaryMinus
  OT3 : Outport  VectorParamsAs1DForOutWhenUnconnected=off
  wires:
  Matrix Concatenate/1 -> OT3/1
  Trigonometric Function7/1 -> Unary Minus/1, Matrix Concatenate2/1
  Unary Minus/1 -> Matrix Concatenate1/2
  psi/1 -> Trigonometric Function/1, Trigonometric Function7/1
  Trigonometric Function/1 -> Matrix Concatenate1/1, Matrix Concatenate2/2
  Matrix Concatenate3/1 -> Matrix Concatenate/3
  Matrix Concatenate2/1 -> Matrix Concatenate/2
  Matrix Concatenate1/1 -> Matrix Concatenate/1
  Constant/1 -> Matrix Concatenate3/1
  Constant1/1 -> Matrix Concatenate3/3
  Constant2/1 -> Matrix Concatenate1/3
  Constant3/1 -> Matrix Concatenate2/3
  Constant4/1 -> Matrix Concatenate3/2

== system ESM_TeslaModelS_statKreisfahrt/Dynamics/SingleTrackModel_linear/vehicle_model/Transformation/trafo_matrix1 ==
  psi : Inport
  Constant{,1,3..4} (4 alike) : Constant  Value=0
  Constant2 : Constant
  Matrix Concatenate : Concatenate  NumInputs=3  Mode=Multidimensional array  ConcatenateDimension=2
  Matrix Concatenate1 : Concatenate  NumInputs=3
  Matrix Concatenate2 : Concatenate  NumInputs=3
  Matrix Concatenate3 : Concatenate  NumInputs=3
  Trigonometric Function : Trigonometry  Operator=cos
  Trigonometric Function7 : Trigonometry
  Unary Minus : UnaryMinus
  OTo : Outport  VectorParamsAs1DForOutWhenUnconnected=off
  wires:
  Constant3/1 -> Matrix Concatenate3/2
  Constant2/1 -> Matrix Concatenate3/1
  Constant1/1 -> Matrix Concatenate2/1
  Constant/1 -> Matrix Concatenate1/1
  Matrix Concatenate1/1 -> Matrix Concatenate/1
  Matrix Concatenate2/1 -> Matrix Concatenate/2
  Matrix Concatenate3/1 -> Matrix Concatenate/3
  Trigonometric Function7/1 -> Matrix Concatenate2/3, Unary Minus/1
  psi/1 -> Trigonometric Function7/1, Trigonometric Function/1
  Unary Minus/1 -> Matrix Concatenate1/2
  Trigonometric Function/1 -> Matrix Concatenate1/3, Matrix Concatenate2/2
  Matrix Concatenate/1 -> OTo/1
  Constant4/1 -> Matrix Concatenate3/3

== system ESM_TeslaModelS_statKreisfahrt/Dynamics/SingleTrackModel_linear/vehicle_model/Transformation1/trafo_matrix ==
  psi : Inport
  Constant{,2..4} (4 alike) : Constant  Value=0
  Constant1 : Constant
  Matrix Concatenate : Concatenate  NumInputs=3  Mode=Multidimensional array  ConcatenateDimension=2
  Matrix Concatenate1 : Concatenate  NumInputs=3
  Matrix Concatenate2 : Concatenate  NumInputs=3
  Matrix Concatenate3 : Concatenate  NumInputs=3
  Trigonometric Function : Trigonometry  Operator=cos
  Trigonometric Function7 : Trigonometry
  Unary Minus4 : UnaryMinus
  OT3 : Outport  VectorParamsAs1DForOutWhenUnconnected=off
  wires:
  Matrix Concatenate1/1 -> Matrix Concatenate/1
  Matrix Concatenate2/1 -> Matrix Concatenate/2
  Trigonometric Function7/1 -> Unary Minus4/1, Matrix Concatenate1/2
  Trigonometric Function/1 -> Matrix Concatenate2/2, Matrix Concatenate1/1
  Matrix Concatenate3/1 -> Matrix Concatenate/3
  Matrix Concatenate/1 -> OT3/1
  Unary Minus4/1 -> Matrix Concatenate2/1
  psi/1 -> Trigonometric Function/1, Trigonometric Function7/1
  Constant/1 -> Matrix Concatenate1/3
  Constant1/1 -> Matrix Concatenate3/3
  Constant2/1 -> Matrix Concatenate2/3
  Constant3/1 -> Matrix Concatenate3/1
  Constant4/1 -> Matrix Concatenate3/2

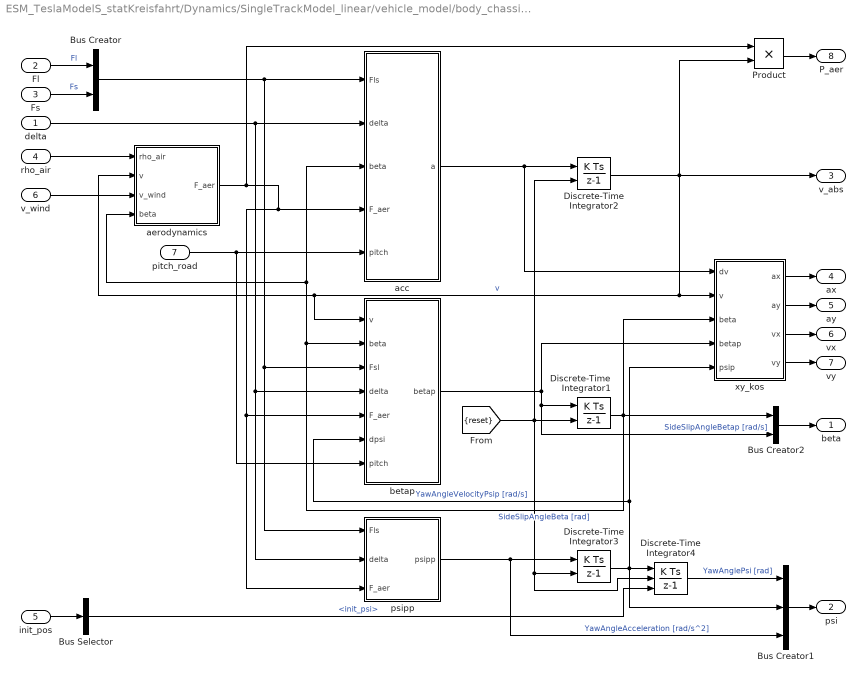
== system ESM_TeslaModelS_statKreisfahrt/Dynamics/SingleTrackModel_linear/vehicle_model/body_chassis_vert/horizontal ==
  delta : Inport
  Fl : Inport  Port=2
  Fs : Inport  Port=3
  rho_air : Inport  Port=4
  init_pos : Inport  Port=5
  v_wind : Inport  Port=6
  pitch_road : Inport  Port=7
  Bus Creator : BusCreator  Inputs=2
  Bus Creator1 : BusCreator  Inputs=3
  Bus Creator2 : BusCreator  Inputs=2
  Bus Selector : BusSelector  OutputSignals=init_psi
  Discrete-Time Integrator1 : DiscreteIntegrator  ExternalReset=sampled level  SampleTime=-1  ICPrevOutput=DiscIntNeverNeededParam  ICPrevScaledInput=DiscIntNeverNeededParam
  Discrete-Time Integrator2 : DiscreteIntegrator  ExternalReset=sampled level  InitialCondition=v0  SampleTime=-1  LimitOutput=on  ICPrevOutput=DiscIntNeverNeededParam  ICPrevScaledInput=DiscIntNeverNeededParam
  Discrete-Time Integrator3 : DiscreteIntegrator  ExternalReset=sampled level  InitialCondition=psip0  SampleTime=-1  ICPrevOutput=DiscIntNeverNeededParam  ICPrevScaledInput=DiscIntNeverNeededParam
  Discrete-Time Integrator4 : DiscreteIntegrator  ExternalReset=sampled level  InitialConditionSource=external  SampleTime=-1  ICPrevOutput=DiscIntNeverNeededParam  ICPrevScaledInput=DiscIntNeverNeededParam
  Product : Product
  acc : Subsystem
  aerodynamics : Subsystem
  betap : Subsystem
  psipp : Subsystem
  xy_kos : Subsystem
  beta : Outport  VectorParamsAs1DForOutWhenUnconnected=off
  psi : Outport  Port=2  VectorParamsAs1DForOutWhenUnconnected=off
  v_abs : Outport  Port=3  VectorParamsAs1DForOutWhenUnconnected=off
  ax : Outport  Port=4  VectorParamsAs1DForOutWhenUnconnected=off
  ay : Outport  Port=5  VectorParamsAs1DForOutWhenUnconnected=off
  vx : Outport  Port=6  VectorParamsAs1DForOutWhenUnconnected=off
  vy : Outport  Port=7  VectorParamsAs1DForOutWhenUnconnected=off
  P_aer : Outport  Port=8  VectorParamsAs1DForOutWhenUnconnected=off
  wires:
  Discrete-Time Integrator2/1 -> v_abs/1, xy_kos/2(v), aerodynamics/2(v), betap/1(v), Product/2  "v"
  Discrete-Time Integrator1/1 -> Bus Creator2/1, aerodynamics/4(beta), acc/3(beta), betap/2(beta), xy_kos/3(beta)  "SideSlipAngleBeta [rad]"
  Bus Creator2/1 -> beta/1
  pitch_road/1 -> betap/7(pitch), acc/5(pitch)
  xy_kos/4(vy) -> vy/1
  xy_kos/2(ay) -> ay/1
  v_wind/1 -> aerodynamics/3(v_wind)
  Bus Selector/1 -> Discrete-Time Integrator4/3  "<init_psi>"
  init_pos/1 -> Bus Selector/1
  [reset] -> Discrete-Time Integrator4/2, Discrete-Time Integrator3/2, Discrete-Time Integrator1/2, Discrete-Time Integrator2/2
  rho_air/1 -> aerodynamics/1(rho_air)
  xy_kos/1(ax) -> ax/1
  Fl/1 -> Bus Creator/1  "Fl"
  Fs/1 -> Bus Creator/2  "Fs"
  Discrete-Time Integrator3/1 -> Discrete-Time Integrator4/1, Bus Creator1/2, xy_kos/5(psip), betap/6(dpsi)  "YawAngleVelocityPsip [rad/s]"
  psipp/1(psipp) -> Discrete-Time Integrator3/1, Bus Creator1/3  "YawAngleAcceleration [rad/s^2]"
  betap/1(betap) -> Bus Creator2/2, Discrete-Time Integrator1/1, xy_kos/4(betap)  "SideSlipAngleBetap [rad/s]"
  delta/1 -> acc/2(delta), psipp/2(delta), betap/4(delta)
  aerodynamics/1(F_aer) -> Product/1, psipp/3(F_aer), betap/5(F_aer), acc/4(F_aer)
  acc/1(a) -> xy_kos/1(dv), Discrete-Time Integrator2/1
  Discrete-Time Integrator4/1 -> Bus Creator1/1  "YawAnglePsi [rad]"
  Bus Creator1/1 -> psi/1
  xy_kos/3(vx) -> vx/1
  Bus Creator/1 -> acc/1(Fls), psipp/1(Fls), betap/3(Fsl)
  Product/1 -> P_aer/1

== system ESM_TeslaModelS_statKreisfahrt/Dynamics/SingleTrackModel_linear/vehicle_model/body_chassis_vert/road_orientation ==
  zroad : Inport
  Bus Selector1 : BusSelector  OutputSignals=zroad_F,zroad_R
  Divide8 : Product  Inputs=*/
  Subtract20 : Sum  Inputs=+-
  Trigonometric Function : Trigonometry  Operator=asin
  theta_road : Outport  VectorParamsAs1DForOutWhenUnconnected=off
  wires:
  Divide8/1 -> Trigonometric Function/1
  [l] -> Divide8/2
  Subtract20/1 -> Divide8/1
  Bus Selector1/1 -> Subtract20/1  "<zroad_F>"
  Trigonometric Function/1 -> theta_road/1
  Bus Selector1/2 -> Subtract20/2  "<zroad_R>"
  zroad/1 -> Bus Selector1/1

== system ESM_TeslaModelS_statKreisfahrt/Dynamics/SingleTrackModel_linear/vehicle_model/body_chassis_vert/transformation ==
  ax : Inport
  ay : Inport  Port=2
  vx : Inport  Port=3
  vy : Inport  Port=4
  Bus Creator1 : BusCreator  Inputs=2
  Bus Creator2 : BusCreator  Inputs=2
  axy : Outport  VectorParamsAs1DForOutWhenUnconnected=off
  vxy : Outport  Port=2  VectorParamsAs1DForOutWhenUnconnected=off
  wires:
  Bus Creator2/1 -> vxy/1
  vy/1 -> Bus Creator2/2  "vy [m/s]"
  vx/1 -> Bus Creator2/1  "vx [m/s]"
  Bus Creator1/1 -> axy/1
  ay/1 -> Bus Creator1/2  "ay [m/s^2]"
  ax/1 -> Bus Creator1/1  "ax [m/s^2]"

== system ESM_TeslaModelS_statKreisfahrt/Dynamics/SingleTrackModel_linear/vehicle_model/body_chassis_vert/vertical ==
  note: Momentengleichgewicht um Vorderrad bzw. Hinterrad --> Vertikalkräfte an Rädern
  Bus Creator1 : BusCreator  Inputs=2
  Divide : Product  Inputs=**/
  Product1 : Product  RndMeth=Zero
  Product3 : Product  RndMeth=Zero
  Signal Conversion2 : SignalConversion  OverrideOpt=off
  Signal Conversion3 : SignalConversion  OverrideOpt=off
  F_vert : Outport  VectorParamsAs1DForOutWhenUnconnected=off
  wires:
  [m] -> Divide/1
  [g] -> Divide/2
  [lR] -> Product3/1
  Bus Creator1/1 -> F_vert/1
  Product3/1 -> Signal Conversion2/1
  Signal Conversion2/1 -> Bus Creator1/1  "F_F"
  Product1/1 -> Signal Conversion3/1
  Signal Conversion3/1 -> Bus Creator1/2  "F_R"
  [l] -> Divide/3
  Divide/1 -> Product1/1, Product3/2
  [lF] -> Product1/2

== system ESM_TeslaModelS_statKreisfahrt/Dynamics/SingleTrackModel_linear/vehicle_model/calc_init/pitch ==
  init_pos : Inport
  Add : Sum
  Add1 : Sum
  Add2 : Sum  Inputs=+-
  Bus Selector : BusSelector  OutputSignals=zroad_RF0,zroad_LF0,zroad_RR0,zroad_LR0
  Divide : Product  Inputs=*/
  Gain : Gain  Gain=0.5
  Gain1 : Gain  Gain=0.5
  Trigonometric Function : Trigonometry  Operator=atan
  init_theta : Outport  VectorParamsAs1DForOutWhenUnconnected=off
  wires:
  Bus Selector/3 -> Add1/1  "<zroad_RR0>"
  Bus Selector/2 -> Add/2  "<zroad_LF0>"
  init_pos/1 -> Bus Selector/1
  Bus Selector/1 -> Add/1  "<zroad_RF0>"
  Add/1 -> Gain/1
  Add1/1 -> Gain1/1
  Bus Selector/4 -> Add1/2  "<zroad_LR0>"
  Gain/1 -> Add2/1
  Gain1/1 -> Add2/2
  Add2/1 -> Divide/1
  Divide/1 -> Trigonometric Function/1
  [l] -> Divide/2
  Trigonometric Function/1 -> init_theta/1

== system ESM_TeslaModelS_statKreisfahrt/Dynamics/SingleTrackModel_linear/vehicle_model/calc_init/vertical ==
  init_pos : Inport
  theta : Inport  Port=2
  Add : Sum
  Add1 : Sum
  Bus Selector : BusSelector  OutputSignals=zroad_RF0,zroad_LF0
  Gain : Gain  Gain=0.5
  Product : Product  RndMeth=Zero
  Trigonometric Function : Trigonometry
  init_z0 : Outport  VectorParamsAs1DForOutWhenUnconnected=off
  wires:
  Add1/1 -> init_z0/1
  Product/1 -> Add1/2
  Trigonometric Function/1 -> Product/2
  theta/1 -> Trigonometric Function/1
  [lF] -> Product/1
  Gain/1 -> Add1/1
  Add/1 -> Gain/1
  Bus Selector/2 -> Add/2  "<zroad_LF0>"
  Bus Selector/1 -> Add/1  "<zroad_RF0>"
  init_pos/1 -> Bus Selector/1

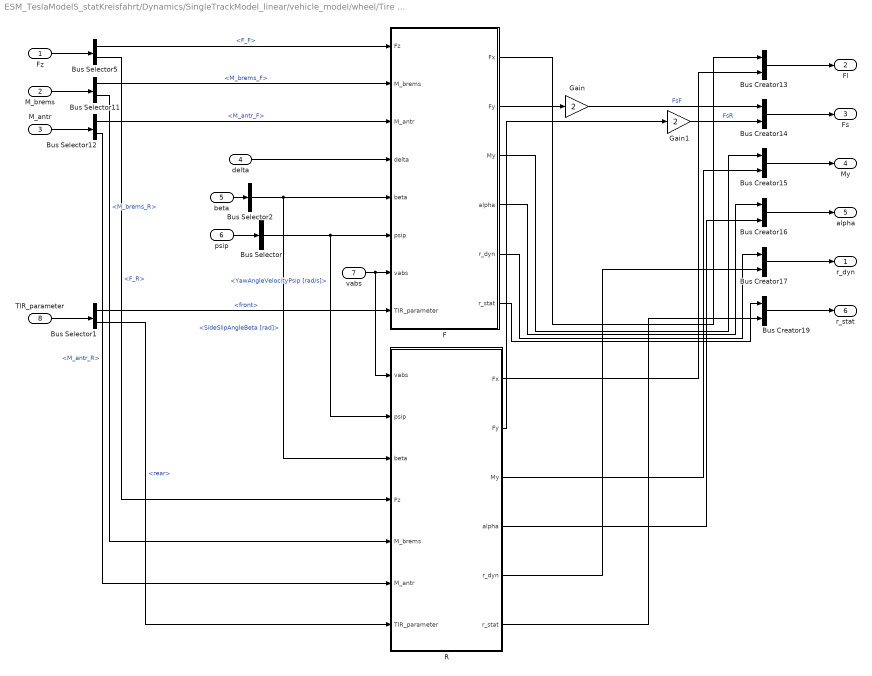
== system ESM_TeslaModelS_statKreisfahrt/Dynamics/SingleTrackModel_linear/vehicle_model/wheel/Tire Model ==
  Fz : Inport
  M_brems : Inport  Port=2
  M_antr : Inport  Port=3
  delta : Inport  Port=4
  beta : Inport  Port=5
  psip : Inport  Port=6
  vabs : Inport  Port=7
  TIR_parameter : Inport  Port=8
  Bus Creator{13..17,19} (6 alike) : BusCreator  Inputs=2
  Bus Selector : BusSelector  OutputSignals=YawAngleVelocityPsip [rad/s]
  Bus Selector1 : BusSelector  OutputSignals=front,rear
  Bus Selector11 : BusSelector  OutputSignals=M_brems_F,M_brems_R
  Bus Selector12 : BusSelector  OutputSignals=M_antr_F,M_antr_R
  Bus Selector2 : BusSelector  OutputSignals=SideSlipAngleBeta [rad]
  Bus Selector5 : BusSelector  OutputSignals=F_F,F_R
  F : Subsystem  mask{mounted_side_input=undefined}
      mask prompts: mounted_side_input "mounted side"
      mask init:
      | switch mounted_side_input
      |     case 1
      |         mounted_side=0;
      |     case 2
      |         mounted_side=1;
      |     case 3
      |         mounted_side=-1;
      | end
      mask TypeOptions mounted_side_input: undefined | left | right
  Gain : Gain  Gain=2
  Gain1 : Gain  Gain=2
  R : Subsystem  mask{mounted_side_input=undefined}
      mask prompts: mounted_side_input "mounted side"
      mask init:
      | switch mounted_side_input
      |     case 1
      |         mounted_side=0;
      |     case 2
      |         mounted_side=1;
      |     case 3
      |         mounted_side=-1;
      | end
      mask TypeOptions mounted_side_input: undefined | left | right
  r_dyn : Outport  VectorParamsAs1DForOutWhenUnconnected=off
  Fl : Outport  Port=2  VectorParamsAs1DForOutWhenUnconnected=off
  Fs : Outport  Port=3  VectorParamsAs1DForOutWhenUnconnected=off
  My : Outport  Port=4  VectorParamsAs1DForOutWhenUnconnected=off
  alpha : Outport  Port=5  VectorParamsAs1DForOutWhenUnconnected=off
  r_stat : Outport  Port=6  VectorParamsAs1DForOutWhenUnconnected=off
  wires:
  Gain1/1 -> Bus Creator14/2  "FsR"
  Gain/1 -> Bus Creator14/1  "FsF"
  beta/1 -> Bus Selector2/1
  psip/1 -> Bus Selector/1
  Fz/1 -> Bus Selector5/1
  Bus Selector5/1 -> F/1(Fz)  "<F_F>"
  Bus Selector5/2 -> R/4(Fz)  "<F_R>"
  F/1(Fx) -> Bus Creator13/1
  R/1(Fx) -> Bus Creator13/2
  Bus Creator14/1 -> Fs/1
  F/2(Fy) -> Gain/1
  R/2(Fy) -> Gain1/1
  F/3(My) -> Bus Creator15/1
  R/3(My) -> Bus Creator15/2
  R/4(alpha) -> Bus Creator16/2
  R/5(r_dyn) -> Bus Creator17/2
  F/5(r_dyn) -> Bus Creator17/1
  Bus Creator15/1 -> My/1
  F/4(alpha) -> Bus Creator16/1
  Bus Creator16/1 -> alpha/1
  Bus Creator17/1 -> r_dyn/1
  Bus Creator19/1 -> r_stat/1
  F/6(r_stat) -> Bus Creator19/1
  R/6(r_stat) -> Bus Creator19/2
  Bus Creator13/1 -> Fl/1
  M_brems/1 -> Bus Selector11/1
  M_antr/1 -> Bus Selector12/1
  Bus Selector11/1 -> F/2(M_brems)  "<M_brems_F>"
  Bus Selector12/1 -> F/3(M_antr)  "<M_antr_F>"
  Bus Selector12/2 -> R/6(M_antr)  "<M_antr_R>"
  Bus Selector11/2 -> R/5(M_brems)  "<M_brems_R>"
  Bus Selector2/1 -> R/3(beta), F/5(beta)  "<SideSlipAngleBeta [rad]>"
  Bus Selector/1 -> R/2(psip), F/6(psip)  "<YawAngleVelocityPsip [rad/s]>"
  vabs/1 -> R/1(vabs), F/7(vabs)
  delta/1 -> F/4(delta)
  TIR_parameter/1 -> Bus Selector1/1
  Bus Selector1/1 -> F/8(TIR_parameter)  "<front>"
  Bus Selector1/2 -> R/7(TIR_parameter)  "<rear>"

== system ESM_TeslaModelS_statKreisfahrt/Dynamics/SingleTrackModel_linear/vehicle_model/wheel/calc_omega ==
  vl : Inport
  r_dyn : Inport  Port=2
  Bus Creator : BusCreator  Inputs=2
  Bus Selector : BusSelector  OutputSignals=vl_F,vl_R
  Bus Selector6 : BusSelector  OutputSignals=r_dyn_F,r_dyn_R
  Divide1 : Product  Inputs=*/
  Divide3 : Product  Inputs=*/
  Unit Delay1 : UnitDelay  InitialCondition=0.3  SampleTime=-1  HasFrameUpgradeWarning=on
  Unit Delay3 : UnitDelay  InitialCondition=0.3  SampleTime=-1  HasFrameUpgradeWarning=on
  omega : Outport  VectorParamsAs1DForOutWhenUnconnected=off
  wires:
  Divide3/1 -> Bus Creator/2  "omega_R"
  Bus Selector/2 -> Divide3/1  "<vl_R>"
  Divide1/1 -> Bus Creator/1  "omega_F"
  Bus Selector/1 -> Divide1/1  "<vl_F>"
  vl/1 -> Bus Selector/1
  Bus Creator/1 -> omega/1
  Unit Delay1/1 -> Divide1/2
  Unit Delay3/1 -> Divide3/2
  r_dyn/1 -> Bus Selector6/1
  Bus Selector6/1 -> Unit Delay1/1  "<r_dyn_F>"
  Bus Selector6/2 -> Unit Delay3/1  "<r_dyn_R>"

== system ESM_TeslaModelS_statKreisfahrt/Dynamics/SingleTrackModel_linear/vehicle_model/wheel/calc_v ==
  delta : Inport
  beta : Inport  Port=2
  psi : Inport  Port=3
  v : Inport  Port=4
  calc_vl : Subsystem
  calc_vs : Subsystem
  vl : Outport  VectorParamsAs1DForOutWhenUnconnected=off
  vs : Outport  Port=2  VectorParamsAs1DForOutWhenUnconnected=off
  wires:
  calc_vs/1(vs) -> vs/1
  beta/1 -> calc_vs/2(beta), calc_vl/4(beta)
  v/1 -> calc_vs/4(v), calc_vl/2(v)
  calc_vl/1(vl) -> vl/1
  [lR] -> calc_vs/6(lR)
  [lF] -> calc_vl/1(lF), calc_vs/5(lF)
  delta/1 -> calc_vs/1(delta), calc_vl/5(delta)
  psi/1 -> calc_vl/3(psi), calc_vs/3(psi)

== system ESM_TeslaModelS_statKreisfahrt/Dynamics/SingleTrackModel_linear/vehicle_model/wheel/v0_korr ==
  vl : Inport
  omega : Inport  Port=2
  r_dyn : Inport  Port=3
  Bus Creator : BusCreator  Inputs=2
  Bus Selector : BusSelector  OutputSignals=vl_F,vl_R
  Bus Selector1 : BusSelector  OutputSignals=r_dyn_F,r_dyn_R
  Bus Selector2 : BusSelector  OutputSignals=omega_F,omega_R
  Subsystem2 : vehicle_model/vehicle_model/wheel/v0_korr/Subsystem4  SystemSampleTime=-1  VariantActivationTime=update diagram  Latency=0  AutoFrameSizeCalculation=off
  Subsystem4 : Subsystem
  v_low : Constant  Value=0.01  VectorParams1D=off
  omega_out : Outport  VectorParamsAs1DForOutWhenUnconnected=off
  wires:
  Subsystem2/1 -> Bus Creator/2  "omega_R [rad/s]"
  Subsystem4/1(omega_out) -> Bus Creator/1  "omega_F [rad/s]"
  Bus Selector2/2 -> Subsystem2/4  "<omega_R>"
  Bus Selector2/1 -> Subsystem4/4(omega)  "<omega_F>"
  Bus Selector1/2 -> Subsystem2/3  "<r_dyn_R>"
  Bus Selector1/1 -> Subsystem4/3(r_dyn)  "<r_dyn_F>"
  v_low/1 -> Subsystem2/2, Subsystem4/2(v_low)
  Bus Selector/2 -> Subsystem2/1  "<vl_R>"
  Bus Selector/1 -> Subsystem4/1(vl)  "<vl_F>"
  Bus Creator/1 -> omega_out/1
  omega/1 -> Bus Selector2/1
  r_dyn/1 -> Bus Selector1/1
  vl/1 -> Bus Selector/1
